simulink model "mpc_pendcartImplicitMPC_nonlinear"  (R2019a)
settings: Solver=ode15s  StartTime=0.0  StopTime=30  MaxStep=1e-3  RelTol=1e-3  EnableMultiTasking=on
values from neighbouring files (symbols this model uses):
  A = [0,1 ... (first row only)    [ControlOfAnInvertedPendulumOnACartExample.m]
  B = [0; (L/J)]    [ControlOfAnInvertedPendulumOnACartExample.m]
  C = [1 0]    [ControlOfAnInvertedPendulumOnACartExample.m]
  D = [0]    [ControlOfAnInvertedPendulumOnACartExample.m]
  f = 1    [ControlOfAnInvertedPendulumOnACartExample.m]
  GoalPos = [pi;0]    [ControlOfAnInvertedPendulumOnACartExample.m]
  J = 1    [ControlOfAnInvertedPendulumOnACartExample.m]
  K = place(A,B,p)    [ControlOfAnInvertedPendulumOnACartExample.m]
  l = 0.45    [ControlOfAnInvertedPendulumOnACartExample.m]
  m_p = 0.853    [ControlOfAnInvertedPendulumOnACartExample.m]
undefined symbols (not defined in the file or in its folder): y0
settings Model: Creator=The MathWorks, Inc.  LastModifiedBy=Lucifer
settings SolverCC: AlgebraicLoopSolver=LineSearch  MinimalZcImpactIntegration=on
settings DataIOCC: LimitDataPoints=on  SaveFormat=Array  ReturnWorkspaceOutputs=off
settings OptimizationCC: LifeSpan=inf
settings DebuggingCC: AlgebraicLoopMsg=none  UnderspecifiedInitializationDetection=Classic  MergeDetectMultiDrivingBlocksExec=none  SolverPrmCheckMsg=warning  AllowSymbolicDim=off  StateNameClashWarn=warning  PregeneratedLibrarySubsystemCodeDiagnostic=none  SFUnexpectedBacktrackingDiag=warning  SFNoUnconditionalDefaultTransitionDiag=warning  SFExecutionAtInitializationDiag=none  ArithmeticOperatorsInVariantConditions=warning
settings HardwareCC: ProdBitPerPointer=32  ProdBitPerSizeT=32  ProdBitPerPtrDiffT=32  ProdLargestAtomicFloat=None  ProdIntDivRoundTo=Undefined  ProdEndianess=Unspecified  ProdWordSize=32  ProdHWDeviceType=32-bit Generic
settings ModelReferenceCC: PropagateSignalLabelsOutOfModel=off
settings SFSimCC: SimUseLocalCustomCode=off
settings RTWCC: RTWUseLocalCustomCode=off
settings CodeAppCC: StateflowObjectComments=on
settings GRTTargetCC: TargetLangStandard=C89/C90 (ANSI)  GeneratePreprocessorConditionals=Disable all
settings ConfigComp: CovMetricSettings=dw  CovHtmlReporting=on  CovSaveCumulativeToWorkspaceVar=on  CovSaveSingleToWorkspaceVar=on  CovExternalEMLEnable=off  CovSFcnEnable=off
settings SimscapeCC: SimscapeNormalizeSystem=off
settings ConfigurationSet: Description=SimMechanics 2G
settings ExplorerConfigSet: InternalSimMechanicsExplorerSettings="<ExplorerConfiguration><canonicalview>default</canonicalview><AnimationSetting><BasePlaybackSpeed>1.0</BasePlaybackSpeed><PlaybackSpeedFactor>1.0</PlaybackSpeedFactor></AnimationSetting><TilePanel><TileInfo><Tiles Columns=\"1\" Count=\"1\" Rows=\"1\"><Column Left=\"2\" Weight=\"1\"/><Column Left=\"1552\"/><Row Top=\"2\" Weight=\"1\"/><Row Top=\"932\"/><Tile Height=\"1\" Width=\"1\" X=\"0\" Y=\"0\"/></Tiles></TileInfo><SceneInfo><SceneViewer><BGColor><R>0.60000002384185791</R><G>0.60000002384185791</G><B>0.60000002384185791</B></BGColor><Camera><Position><X>0.027865189060748197</X><Y>-2.5719092456962986</Y><Z>0.23157896538506753</Z></Position><Center><X>0.62659712312732463</X><Y>-0.46110119691712204</Y><Z>0.22087365386473376</Z></Center><Up><X>-0.0079438354874226333</X><Y>0.0073246425924307582</Y><Z>0.99994162084025784</Z></Up><Left>-0.24533778208815546</Left><Right>0.24533778208815546</Right><Bottom>-0.79734779727023208</Bottom><Top>0.79734779727023208</Top></Camera></SceneViewer></SceneInfo></TilePanel></ExplorerConfiguration>"

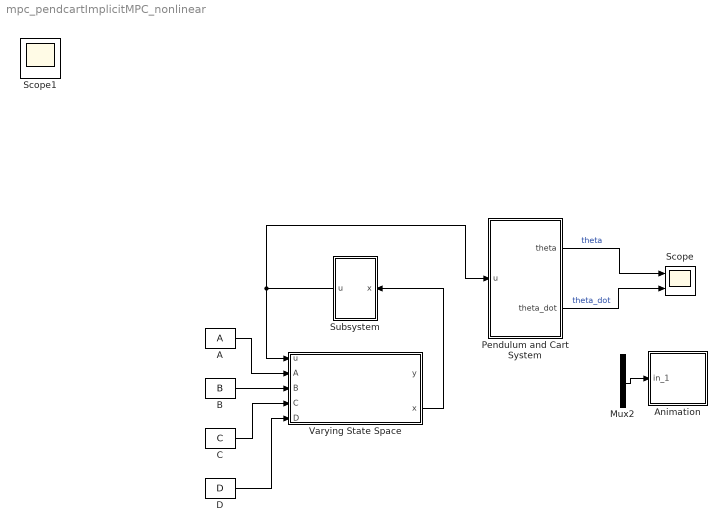
== system mpc_pendcartImplicitMPC_nonlinear ==
  A : Constant  Value=A
  Animation : Subsystem  mask(Pendulum plot){RefBlock=x Ref}
      mask prompts: RefBlock "Cart Reference Signal Block Name:"
      mask help: Pendulum plot
      mask Help: Pendulum animation function using Handle graphics.
      mask Display: plot([-10 10],[0 0],[-2 -2 2 2],[0 1 1 0],[0 3],[1 5])
  B : Constant  Value=B
  C : Constant  Value=C
  D : Constant  Value=D
  Mux2 : Mux  Inputs=2
  Pendulum and Cart System : Subsystem  mask{mCartPara=1, mPendPara=1, gPara=9.81, LPara=0.5, KdPara=10}
      mask prompts: mCartPara "Mass of Cart"; mPendPara "Mass of Pendulum"; gPara "Gravity"; LPara "Length of Pendulum"; KdPara "Friction coefficient of Cart"
      mask help: Pendulum and Cart System
      mask init:
      | mCart = str2double(get_param(gcb,'mCartPara'));
      | mPend = str2double(get_param(gcb,'mPendPara'));
      | g = str2double(get_param(gcb,'gPara'));
      | L = str2double(get_param(gcb,'LPara'));
      | Kd = str2double(get_param(gcb,'KdPara'));
  Scope : Scope  NumInputPorts=2
  Subsystem : Subsystem
  Varying State Space : Subsystem  AncestorBlock=cstblocks/Linear Parameter Varying/Varying State Space  mask(Varying State Space){x0=y0, xNames='angle', OutputX=on, OutputDX=on}
      mask prompts: x0 "Control:simulink:VaryingSSLabel1"; xNames "Control:simulink:VaryingSSLabel2"; OutputX "Control:simulink:VaryingSSLabel3"; OutputDX "Control:simulink:VaryingSSLabel4"
      mask help: Control:simulink:VaryingSS1
      mask init:
      | % Use exact linearization of product block
      | % pblks = find_system(gcb,'FollowLinks','on',...
      | %    'LookUnderMasks','all','SearchDepth',1,'BlockType','Product');
      | % rep = struct(...
      | %    'Specification','controllib.internal.blocks.matrixProductJacobian',...
      | %    'Type','Function',...
      | %    'ParameterNames','',...
      | %    'ParameterValues','');
      | % for i=1:numel(pblks)
      | %    set_param(pblks{i},...
      | %       'SCDEnableBlockLinearizationSpecification','on',...
      | %       'SCDBlockLinearizationSpecification',rep)
      | % end
      | SimStatus = get_param(bdroot,'SimulationStatus');
      | if any(strcmp(SimStatus,{'initializing','updating','stopped'}))
      |    varyingBlockMask('ss',gcb,OutputX,OutputDX)
      | end
      mask Help: eval('ctrlguihelp(''VaryingSSCT'');')
      mask DialogControl x0 Prompt: Initial conditions:
      mask DialogControl xNames Prompt: State names (e.g., 'position'):
      mask DialogControl OutputX Prompt: Output states
      mask DialogControl OutputDX Prompt: Output state derivatives
      mask Display:
      | port_label('input', 1, 'u')
      | port_label('input', 2, 'A')
      | port_label('input', 3, 'B')
      | port_label('input', 4, 'C')
      | port_label('input', 5, 'D')
      | port_label('output', 1, 'y')
      | next_ = 2;
      | if OutputX
      |    port_label('output', next_, 'x')
      |    next_ = next_+1;
      | end
      | if OutputDX
      |    port_label('output', next_, 'dx')
      |    next_ = next_+1;
      | end
      | text(0.5,0.65,'dx = A x + B u',...
      |    'horizontalAlignment', 'center','texmode','on')
      | text(0.5,0.35,'y = C x + D u',...
      |    'horizontalAlignment', 'center','texmode','on')
  Scope1 : Scope
  wires:
  A/1 -> Varying State Space/2(A)
  Mux2/1 -> Animation/1(in_1)
  Pendulum and Cart System/2(theta_dot) -> Scope/2  "theta_dot"
  Pendulum and Cart System/1(theta) -> Scope/1  "theta"
  B/1 -> Varying State Space/3(B)
  C/1 -> Varying State Space/4(C)
  D/1 -> Varying State Space/5(D)
  Subsystem/1(u) -> Varying State Space/1(u), Pendulum and Cart System/1(u)
  Varying State Space/2(x) -> Subsystem/1(x)

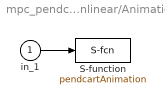
== system mpc_pendcartImplicitMPC_nonlinear/Animation ==
  in_1 : Inport
  S-function : S-Function  FunctionName=pendcartAnimation  Parameters=RefBlock  SFunctionDeploymentMode=off  EnableBusSupport=off
      settings: DeleteFcn=pendcartAnimation([],[],[],'DeleteBlock');
  wires:
  in_1/1 -> S-function/1

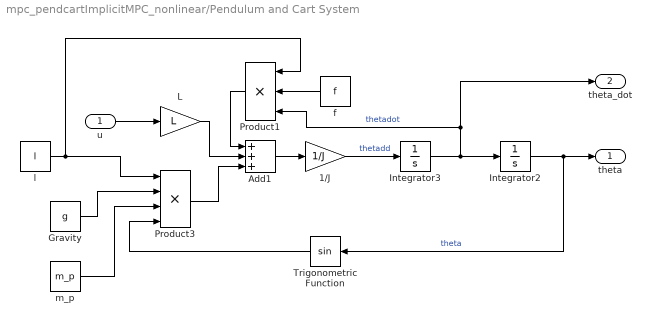
== system mpc_pendcartImplicitMPC_nonlinear/Pendulum and Cart System ==
  u : Inport
  1/J : Gain  Gain=1/J
  Add1 : Sum  Inputs=+++
  Gravity : Constant  Value=g
  Integrator2 : Integrator  ContinuousStateAttributes='theta'
  Integrator3 : Integrator  ContinuousStateAttributes='thetadot'
  L : Gain  Gain=L
  Product1 : Product  Inputs=3
  Product3 : Product  Inputs=4
  Trigonometric Function : Trigonometry
  f : Constant  Value=f
  l : Constant  Value=l
  m_p : Constant  Value=m_p
  theta : Outport
  theta_dot : Outport  Port=2
  wires:
  1/J/1 -> Integrator3/1  "thetadd"
  Product3/1 -> Add1/3
  Integrator3/1 -> Integrator2/1, Product1/3, theta_dot/1  "thetadot"
  Integrator2/1 -> Trigonometric Function/1, theta/1  "theta"
  Add1/1 -> 1/J/1
  L/1 -> Add1/2
  u/1 -> L/1
  l/1 -> Product1/1, Product3/1
  Gravity/1 -> Product3/2
  m_p/1 -> Product3/3
  Trigonometric Function/1 -> Product3/4
  f/1 -> Product1/2
  Product1/1 -> Add1/1

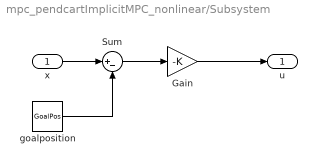
== system mpc_pendcartImplicitMPC_nonlinear/Subsystem ==
  x : Inport
  Gain : Gain  Gain=-K
  Sum : Sum  Inputs=|+-
  goalposition : Constant  Value=GoalPos
  u : Outport
  wires:
  x/1 -> Sum/1
  Gain/1 -> u/1
  Sum/1 -> Gain/1
  goalposition/1 -> Sum/2

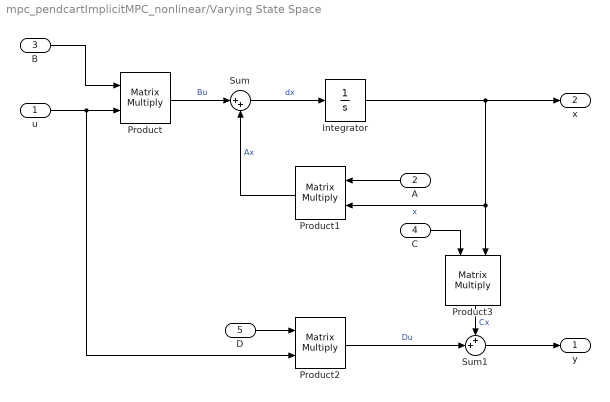
== system mpc_pendcartImplicitMPC_nonlinear/Varying State Space ==
  u : Inport
  A : Inport  Port=2
  B : Inport  Port=3
  C : Inport  Port=4
  D : Inport  Port=5
  Integrator : Integrator  InitialCondition=x0  ContinuousStateAttributes=xNames
  Product{,1..3} (4 alike) : Product  SCDEnableBlockLinearizationSpecification=on  Multiplication=Matrix(*)
  Sum : Sum  Inputs=|++
  Sum1 : Sum  Inputs=++|
  y : Outport
  x : Outport  Port=2
  wires:
  C/1 -> Product3/1
  D/1 -> Product2/1
  u/1 -> Product2/2, Product/2
  A/1 -> Product1/1
  Product1/1 -> Sum/2  "Ax"
  B/1 -> Product/1
  Sum1/1 -> y/1
  Integrator/1 -> x/1, Product1/2, Product3/2  "x"
  Product2/1 -> Sum1/2  "Du"
  Product3/1 -> Sum1/1  "Cx"
  Sum/1 -> Integrator/1  "dx"
  Product/1 -> Sum/1  "Bu"
